simulink model "Main_Firmware_LOCAL"  (R2024b)
settings: Solver=FixedStepDiscrete  StartTime=0.0  StopTime=inf  FixedStep=sample_time  RelTol=1e-3  EnableMultiTasking=on
values from neighbouring files (symbols this model uses):
  A_f = 1.24    [Minh_Inverter_Init.m]
  C_d = 0.7041    [Minh_Inverter_Init.m]
  C_rr = 0.02    [Minh_Inverter_Init.m]
  Current_max = min(InvCurr_RMS,mCurr_RMS)*sqrt(2)    [Minh_Inverter_Init.m]
  Encoder_Offset = (PhaseA_offset/ppair)*pi/180    (= -0.785398163397)    [Minh_Inverter_Init.m]
  EPWM_F = 200000    [Minh_Inverter_Init.m]
  g = 9.8    [Minh_Inverter_Init.m]
  Inertia_z = c2d(Inertia_s, sample_time, 'zoh')    [Minh_Inverter_Init.m]
  k = 1    [Minh_Inverter_Init.m]
  lambda = 0.0375    [Minh_Inverter_Init.m]
  Ld = 0.1e-3    (= 0.0001)    [Minh_Inverter_Init.m]
  Lq = Ld    (= 0.0001)    [Minh_Inverter_Init.m]
  m = 1    [Minh_Inverter_Init.m]
  ppair = 4    [Minh_Inverter_Init.m]
  r = 0.4064/2    (= 0.2032)    [Minh_Inverter_Init.m]
  rho = 1.2    [Minh_Inverter_Init.m]
  Rs = (Rpp^2)/(Rpp*3)    (= 0.00433333333333)    [Minh_Inverter_Init.m]
  sample_time = 1/10000    (= 0.0001)    [Minh_Inverter_Init.m]
  speed_max = rpm_max*2*pi/60    (= 523.598775598)    [Minh_Inverter_Init.m]
  Torque_max = Current_max*3*lambda*ppair/2    [Minh_Inverter_Init.m]
  Voltage_max = min(V_dd,mVolt_RMS*sqrt(2))    [Minh_Inverter_Init.m]
undefined symbols (not defined in the file or in its folder): DiscIntNeverNeededParam, dspblkCoreblockFVToolHelper, gcbh, GPTRIP1SEL, TZ1
libraries: c2802xlib x8, simulink x4, slpidlib x3, spsabctodq0Lib x2, c28004xlib x1, spsdq0toabcLib x1
(part 1 of 2)
settings Model: SimulationMode=external  ExtModeTrigDuration=8  Creator=minhp  LastModifiedBy=minhp
settings SolverCC: AllowMultiTaskInputOutput=on  AutoInsertRateTranBlk=on
settings OptimizationCC: DefaultUnderspecifiedDataType=single  EnhancedBackFolding=on  PassReuseOutputArgsAs=Individual arguments  MaxStackSize=1024  OptimizeBlockOrder=speed  DifferentSizesBufferReuse=on  OptimizationCustomize=off  EfficientTunableParamExpr=on
settings DebuggingCC: SingleTaskRateTransMsg=warning  IntegerOverflowMsg=error  ParameterTunabilityLossMsg=error  IntegerSaturationMsg=error
settings HardwareCC: ProdBitPerChar=16  ProdBitPerInt=16  ProdBitPerPointer=32  ProdBitPerSizeT=32  ProdBitPerPtrDiffT=32  ProdLargestAtomicInteger=Integer  ProdLargestAtomicFloat=None  ProdWordSize=16  ProdLongLongMode=on  ProdHWDeviceType=Texas Instruments->C2000  HardwareBoardFeatureSet=SoCBlockset
settings SFSimCC: MATLABDynamicMemAlloc=off
settings RTWCC: Description=Embedded Coder  SystemTargetFile=ert.tlc  HardwareBoard=TI Piccolo F280049C LaunchPad  TemplateMakefile=ert_default_tmf  Toolchain=Texas Instruments Code Composer Studio (C2000)  CodeProfilingSaveOptions=MetricsOnly
settings CodeAppCC: ForceParamTrailComments=on  IgnoreCustomStorageClasses=off  OperatorAnnotations=on  SimulinkDataObjDesc=on  SFDataObjDesc=on  InsertBlockDesc=on
settings ERTTargetCC: CodeReplacementLibrary=TI C28x  SupportContinuousTime=on  ExtModeTransport=4  ExtModeStaticAlloc=on  ExtModeAutomaticAllocSize=off  ExtModeStaticAllocSize=5000  ExtModeMexFile=ext_xcp  ExtModeIntrfLevel=Level2 - Open  InlinedParameterPlacement=Hierarchical  DynamicArrayContainerType=coder::array

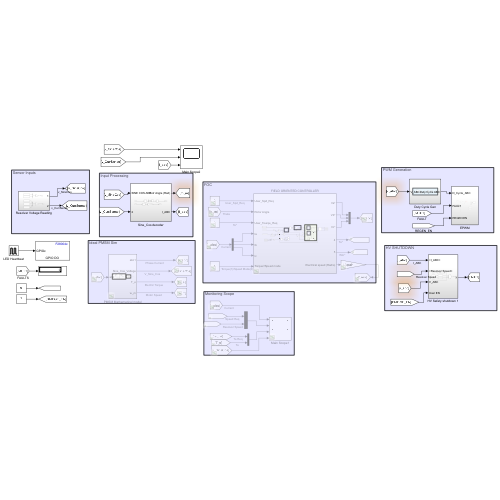
[thumbnail: Simulink's stored preview of the top-level diagram]
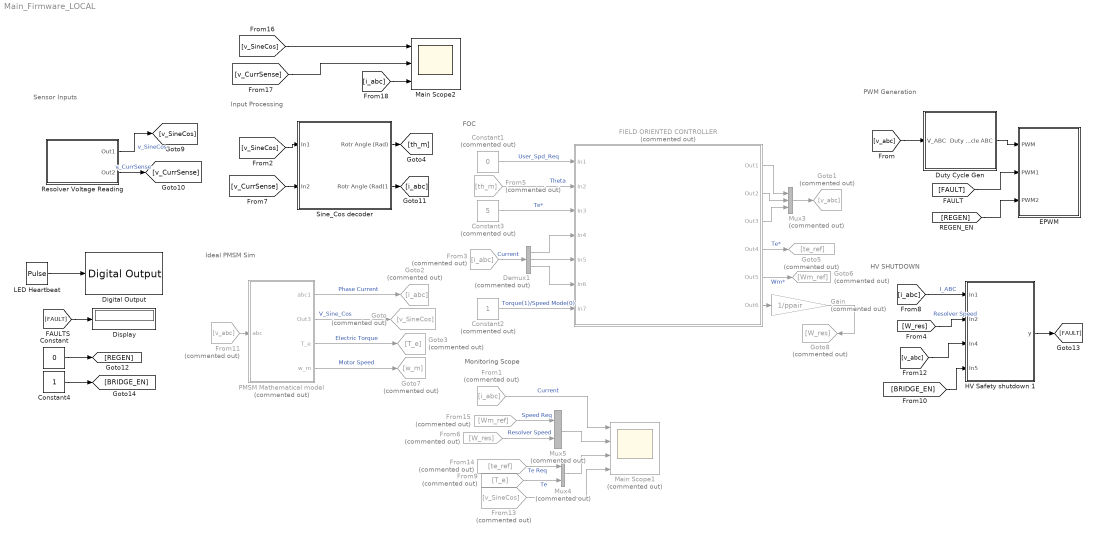
== system Main_Firmware_LOCAL ==
  note: Ideal PMSM Sim
  note: Monitoring Scope
  note: PWM Generation
  note: Input Processing
  note: FOC
  note: Sensor Inputs
  note: HV SHUTDOWN
  Constant : Constant  Value=0
  Constant1 : Constant  Commented=on  Value=0  OutDataTypeStr=single
  Constant2 : Constant  Commented=on
  Constant3 : Constant  Commented=on  Value=5  OutDataTypeStr=single
  Constant4 : Constant
  Demux1 : Demux  Commented=on  Outputs=3
  Digital Output : c28004xlib/Digital Output  GPIO_Number=GPIO16~GPIO23  GPIO_Bit0=off  GPIO_BIT0_Toggle=off  GPIO_Bit1=off  GPIO_BIT1_Toggle=off  GPIO_Bit2=off  GPIO_BIT2_Toggle=off  GPIO_Bit3=off  GPIO_BIT3_Toggle=off  GPIO_Bit4=off  GPIO_BIT4_Toggle=off  GPIO_Bit5=off  GPIO_BIT5_Toggle=off  GPIO_Bit6=off  GPIO_BIT6_Toggle=off  GPIO_Bit7=on  GPIO_BIT7_Toggle=off
  Display : Display
  Duty Cycle Gen : Subsystem
  EPWM : Subsystem
  FIELD ORIENTED CONTROLLER : Subsystem  Commented=on
  From1 : From  Commented=on  GotoTag=i_abc
  From11 : From  Commented=on  GotoTag=v_abc
  From13 : From  Commented=on  GotoTag=v_SineCos
  From14 : From  Commented=on  GotoTag=te_ref
  From15 : From  Commented=on  GotoTag=Wm_ref
  From3 : From  Commented=on  GotoTag=i_abc
  From5 : From  Commented=on  GotoTag=th_m
  From6 : From  Commented=on  GotoTag=W_res
  From9 : From  Commented=on  GotoTag=T_e
  Gain : Gain  Commented=on  Gain=1/ppair
  Goto : Goto  Commented=on  GotoTag=v_SineCos
  Goto1 : Goto  Commented=on  GotoTag=v_abc
  Goto2 : Goto  Commented=on  GotoTag=i_abc
  Goto3 : Goto  Commented=on  GotoTag=T_e
  Goto5 : Goto  Commented=on  GotoTag=te_ref
  Goto6 : Goto  Commented=on  GotoTag=Wm_ref
  Goto7 : Goto  Commented=on  GotoTag=w_m
  Goto8 : Goto  Commented=on  GotoTag=W_res
  HV Safety shutdown 1 : Subsystem
  LED Heartbeat : DiscretePulseGenerator  PulseType=Time based  Period=1  PulseWidth=50
  Main Scope1 : Scope  Commented=on  NumInputPorts=4
  Main Scope2 : Scope  NumInputPorts=3
  Mux3 : Mux  Commented=on  Inputs=3
  Mux4 : Mux  Commented=on  Inputs=2
  Mux5 : Mux  Commented=on  Inputs=2
  PMSM Mathematical model : Subsystem  Commented=on
  Resolver Voltage Reading : Subsystem
  Sine_Cos decoder : Subsystem
  wires:
  Duty Cycle Gen/1(Duty Cycle ABC) -> EPWM/1(PWM)
  PMSM Mathematical model/2(Out3) -> Goto/1  "V_Sine_Cos"
  PMSM Mathematical model/4(w_m) -> Goto7/1  "Motor Speed"
  From11/1 -> PMSM Mathematical model/1(abc)
  PMSM Mathematical model/1(abc1) -> Goto2/1  "Phase Current"
  PMSM Mathematical model/3(T_e) -> Goto3/1  "Electric Torque"
  Constant3/1 -> FIELD ORIENTED CONTROLLER/3(In3)  "Te*"
  FIELD ORIENTED CONTROLLER/1(Out1) -> Mux3/1
  FIELD ORIENTED CONTROLLER/4(Out4) -> Goto5/1  "Te*"
  FIELD ORIENTED CONTROLLER/2(Out2) -> Mux3/2
  FIELD ORIENTED CONTROLLER/3(Out3) -> Mux3/3
  From3/1 -> Demux1/1  "Current"
  From5/1 -> FIELD ORIENTED CONTROLLER/2(In2)  "Theta"
  Demux1/2 -> FIELD ORIENTED CONTROLLER/5(In5)
  Demux1/3 -> FIELD ORIENTED CONTROLLER/6(In6)
  Constant2/1 -> FIELD ORIENTED CONTROLLER/7(In7)  "Torque(1)/Speed Mode(0)"
  Demux1/1 -> FIELD ORIENTED CONTROLLER/4(In4)
  Constant1/1 -> FIELD ORIENTED CONTROLLER/1(In1)  "User_Spd_Req"
  FIELD ORIENTED CONTROLLER/5(Out5) -> Goto6/1  "Wm*"
  [v_abc] -> Duty Cycle Gen/1(V_ABC)
  From6/1 -> Mux5/2  "Resolver Speed"
  From14/1 -> Mux4/1  "Te Req"
  From9/1 -> Mux4/2  "Te"
  Mux5/1 -> Main Scope1/2
  From15/1 -> Mux5/1  "Speed Req"
  From1/1 -> Main Scope1/1  "Current"
  Mux4/1 -> Main Scope1/3
  Mux3/1 -> Goto1/1
  [v_SineCos] -> Sine_Cos decoder/1(In1)
  Sine_Cos decoder/1(Rotr Angle (Rad)) -> [th_m]
  FIELD ORIENTED CONTROLLER/6(Out6) -> Gain/1
  Gain/1 -> Goto8/1
  Resolver Voltage Reading/1(Out1) -> [v_SineCos]  "v_SineCos"
  LED Heartbeat/1 -> Digital Output/1
  Resolver Voltage Reading/2(Out2) -> [v_CurrSense]  "v_CurrSense"
  [v_CurrSense] -> Sine_Cos decoder/2(In2)
  Sine_Cos decoder/2(Rotr Angle (Rad)1) -> [i_abc]
  [FAULT] -> EPWM/2(PWM1)
  [i_abc] -> HV Safety shutdown 1/1(In1)  "I_ABC"
  HV Safety shutdown 1/1(y) -> [FAULT]
  [FAULT] -> Display/1
  [W_res] -> HV Safety shutdown 1/2(In2)  "Resolver Speed"
  [v_abc] -> HV Safety shutdown 1/3(In4)
  From13/1 -> Main Scope1/4
  [v_SineCos] -> Main Scope2/1
  [v_CurrSense] -> Main Scope2/2
  [i_abc] -> Main Scope2/3
  [REGEN] -> EPWM/3(PWM2)
  [BRIDGE_EN] -> HV Safety shutdown 1/4(In5)
  Constant/1 -> [REGEN]
  Constant4/1 -> [BRIDGE_EN]

== system Main_Firmware_LOCAL/Duty Cycle Gen ==
  note: PWM Duty Cycle Generation:
  V_ABC : Inport
  Constant7 : Constant  Value=0.5
  Gain5 : Gain  Gain=1/Voltage_max  OutDataTypeStr=single  RndMeth=Nearest
  Sampling Delay : Delay  DelayLength=1
  Saturation : Saturate  UpperLimit=95  LowerLimit=0  OutDataTypeStr=single  RndMeth=Nearest
  Sum : Sum  Inputs=|++
  Duty Cycle ABC : Outport
  wires:
  Sampling Delay/1 -> Saturation/1
  Gain5/1 -> Sum/1
  Saturation/1 -> Duty Cycle ABC/1
  V_ABC/1 -> Gain5/1
  Constant7/1 -> Sum/2
  Sum/1 -> Sampling Delay/1

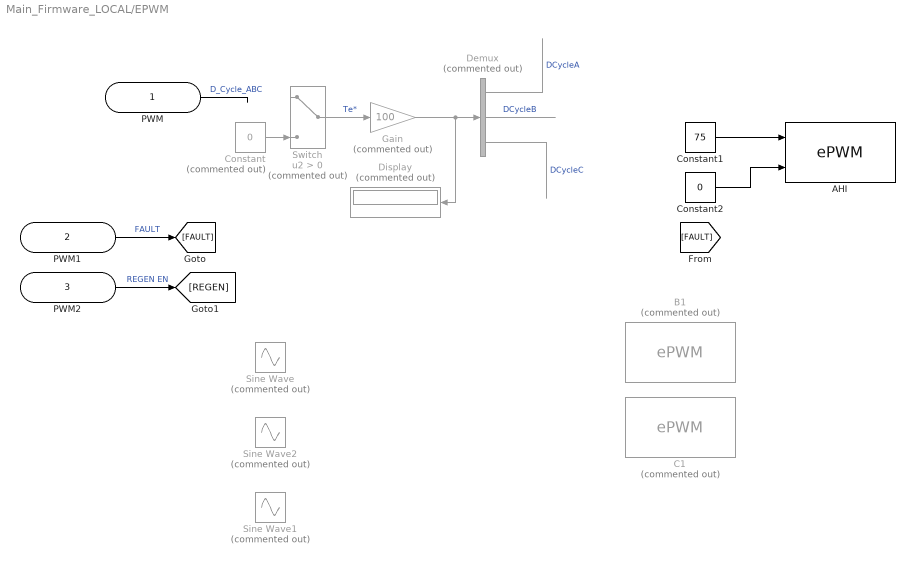
== system Main_Firmware_LOCAL/EPWM ==
  PWM : Inport
  PWM1 : Inport  Port=2
  PWM2 : Inport  Port=3
  AHI : c2802xlib/ePWM  PwmType=C2000_Type4  useModule=ePWM1  ePWMxLINKTBPRD=Not Linked  periodUnits=Seconds  timerSource=Specify via dialog  timerPeriod_clk=1/EPWM_F  timerPeriod_sec=1/EPWM_F  tbshadow=Counter equals to zero  countingMode=Up  phaseActiveEnable=Disable  phaseDirection=Count down after sync  phaseActive=0  synchronizationEnable=off  dcaevt1Sync=off  dcbevt1Sync=off  synchronizationOption=Disable  dcbevt1SyncOut=off  dcaevt1SyncOut=off  cmpdSyncOut=off  cmpcSyncOut=off  cmpbSyncOut=off  zeroSyncOut=off  swfSyncOut=off  perSynchronizationOption=Counter equals to period (CTR=PRD)  clockPrescale=1  HSclockPrescale=1  enswap=off  ePWMxAStatus=on  ePWMxAactionLogic1=Set  ePWMxAactionLogic2=Clear  ePWMxAactionLogic3=Clear  ePWMxAactionLogic4=Set  ePWMxAactionLogic5=Do nothing  ePWMxAactionLogic6=Do nothing  ePWMxACSFenable=on  ePWMxACSFvalue=Forcing low  ePWMxASFreload=Zero  ePWMxBStatus=on  ePWMxBactionLogic1=Set  ePWMxBactionLogic2=Clear  ePWMxBactionLogic3=Clear  ePWMxBactionLogic4=Do nothing  ePWMxBactionLogic5=Do nothing  ePWMxBactionLogic6=Set  ePWMxBCSFenable=off  ePWMxBCSFvalue=Forcing disable  ePWMxBSFreload=Zero  ePWNxBOutWay=off  ePWMxLINKCMPA=Not Linked  CMPAUnits=Percentages  CMPASource=Input port  CMPAValue_per=0  CMPAValue_clk=0  enCMPAshadow=Counter equals to zero (CTR=Zero)  ePWMxLINKCMPB=Not Linked  CMPBUnits=Clock cycles  CMPBSource=Specify via dialog  CMPBValue_per=50  CMPBValue_clk=32000  enCMPBshadow=Counter equals to zero (CTR=Zero)  ePWMxLINKCMPC=Not Linked  CMPCUnits=Percentages  CMPCSource=Specify via dialog  CMPCValue_per=60  CMPCValue_clk=50  enCMPCshadow=Counter equals to zero (CTR=Zero)  ePWMxLINKCMPD=Not Linked  CMPDUnits=Clock cycles  CMPDSource=Specify via dialog  CMPDValue_per=50  CMPDValue_clk=32000  enCMPDshadow=Counter equals to zero (CTR=Zero)  enableDBePWMxA=off  enableDBePWMxB=off  enhalfcycle=off  DBpolarity=Active high (AH)  DBedgeDelay=Positive  DBSource_ePWMxA=ePWMxA  DBSource_ePWMxB=ePWMxA  DBPeriodUnits=Clock cycles  DBperiodSource=Specify via dialog  REDperiod=0  FEDperiod=0  REDperiod_sec=0  FEDperiod_sec=0  LoadModeDBRED=Immediate without using shadow  LoadModeDBFED=Immediate without using shadow  adcstartModuleA=off  adcrequestEventA=First event  adcstartEventA=Digital Compare Module A Event 1 start of conversion (DCAEVT1.soc)  adcstartEventA_type2=Counter equals to zero (CTR=Zero)  adcstartModuleB=off  adcrequestEventB=First event  adcstartEventB=Counter equals to zero (CTR=Zero)  adcstartEventB_type2=Counter equals to zero (CTR=Zero)  intEn=off  intPrd=First event  intSel=Counter equals to zero (CTR=Zero)  intSel_type2=Counter equals to zero (CTR=Zero)  hrpe=off  enHRPWM=off  HRPWM_LoadMode=Counter equals to period (CTR=PRD)  HRPWM_CTLMode=Duty or Period control mode  HRPWM_EDGMode=Both edge  hrpeb=off  enHRPWMB=off  HRPWM_LoadModeB=Counter equals to zero (CTR=ZERO)  HRPWM_CTLModeB=Duty or Period control mode  HRPWM_EDGModeB=Both edge  enHRDBRED=off  enHRDBFED=off  enSFO=on  enautoconv=on  chopperEnable=off  chopperFrequency=1  chopperFirstwidth=1  chopperDuty=12.5%  tripZonesource=Specify via dialog  tzselOSHT1=off  tzselOSHT2=off  tzselOSHT3=off  tzselOSHT4=off  tzselOSHT5=off  tzselOSHT6=off  tzselOSHDCAEV1=off  tzselOSHDCBEV1=off  tzselCBC1=off  tzselCBC2=off  tzselCBC3=off  tzselCBC4=off  tzselCBC5=off  tzselCBC6=off  tzselCBCDCAEV2=off  tzselCBCDCBEV2=off  enTzOstIntr=off  enTzCbcIntr=off  enTzDCAEVT1Intr=off  enTzDCAEVT2Intr=off  enTzDCBEVT1Intr=off  enTzDCBEVT2Intr=off  tzclrCBCLatch=Counter equals to zero (CTR=Zero)  ePWMxAforced=No action  ePWMxBforced=No action  DCAEVT1forced=No action  DCBEVT1forced=No action  DCAEVT2forced=No action  DCBEVT2forced=No action  dcah=Trip Zone 1 input (TZ1)  dcal=Trip Zone 2 input (TZ2)  dcbh=Trip Zone 1 input (TZ1)  dcbl=Trip Zone 2 input (TZ2)  dcah_type2=GPTRIP1SEL/(TZ1)  dcal_type2=GPTRIP1SEL/(TZ1)  dcbh_type2=GPTRIP1SEL/(TZ1)  dcbl_type2=GPTRIP1SEL/(TZ1)  gendcaevt1=Event disabled  gendcaevt2=Event disabled  gendcbevt1=Event disabled  gendcbevt2=Event disabled  dcaevt1src=DCAEVT1 with sync  dcaevt2src=DCAEVT2 with sync  dcbevt1src=DCBEVT1 with sync  dcbevt2src=DCBEVT2 with sync  pulsesel=Counter equals to zero (CTR=Zero)  blankinv=off  blankoffset=0  blankwidth=0  evsrcsel=Filtered version of DCAEVT1 (DCAEVT1FILT)  encape=off
      settings: LibrarySourceBlock=c28004xlib/ePWM
  B1 : c2802xlib/ePWM  Commented=on  PwmType=C2000_Type4  useModule=ePWM4  ePWMxLINKTBPRD=ePWM1  periodUnits=Seconds  timerSource=Specify via dialog  timerPeriod_clk=1/EPWM_F  timerPeriod_sec=1/EPWM_F  tbshadow=Counter equals to zero  countingMode=Up  phaseActiveEnable=Disable  phaseDirection=Count down after sync  phaseActive=0  synchronizationEnable=off  dcaevt1Sync=off  dcbevt1Sync=off  synchronizationOption=Disable  dcbevt1SyncOut=off  dcaevt1SyncOut=off  cmpdSyncOut=off  cmpcSyncOut=off  cmpbSyncOut=off  zeroSyncOut=off  swfSyncOut=off  perSynchronizationOption=Counter equals to period (CTR=PRD)  clockPrescale=1  HSclockPrescale=1  enswap=off  ePWMxAStatus=on  ePWMxAactionLogic1=Set  ePWMxAactionLogic2=Clear  ePWMxAactionLogic3=Clear  ePWMxAactionLogic4=Set  ePWMxAactionLogic5=Do nothing  ePWMxAactionLogic6=Do nothing  ePWMxACSFenable=off  ePWMxACSFvalue=Forcing disable  ePWMxASFreload=Zero  ePWMxBStatus=on  ePWMxBactionLogic1=Set  ePWMxBactionLogic2=Clear  ePWMxBactionLogic3=Clear  ePWMxBactionLogic4=Do nothing  ePWMxBactionLogic5=Do nothing  ePWMxBactionLogic6=Set  ePWMxBCSFenable=off  ePWMxBCSFvalue=Forcing disable  ePWMxBSFreload=Zero  ePWNxBOutWay=off  ePWMxLINKCMPA=Not Linked  CMPAUnits=Percentages  CMPASource=Input port  CMPAValue_per=0  CMPAValue_clk=0  enCMPAshadow=Counter equals to zero (CTR=Zero)  ePWMxLINKCMPB=Not Linked  CMPBUnits=Clock cycles  CMPBSource=Specify via dialog  CMPBValue_per=50  CMPBValue_clk=32000  enCMPBshadow=Counter equals to zero (CTR=Zero)  ePWMxLINKCMPC=Not Linked  CMPCUnits=Percentages  CMPCSource=Specify via dialog  CMPCValue_per=60  CMPCValue_clk=50  enCMPCshadow=Counter equals to zero (CTR=Zero)  ePWMxLINKCMPD=Not Linked  CMPDUnits=Clock cycles  CMPDSource=Specify via dialog  CMPDValue_per=50  CMPDValue_clk=32000  enCMPDshadow=Counter equals to zero (CTR=Zero)  enableDBePWMxA=off  enableDBePWMxB=off  enhalfcycle=off  DBpolarity=Active high (AH)  DBedgeDelay=Positive  DBSource_ePWMxA=ePWMxA  DBSource_ePWMxB=ePWMxA  DBPeriodUnits=Clock cycles  DBperiodSource=Specify via dialog  REDperiod=0  FEDperiod=0  REDperiod_sec=0  FEDperiod_sec=0  LoadModeDBRED=Immediate without using shadow  LoadModeDBFED=Immediate without using shadow  adcstartModuleA=off  adcrequestEventA=First event  adcstartEventA=Digital Compare Module A Event 1 start of conversion (DCAEVT1.soc)  adcstartEventA_type2=Counter equals to zero (CTR=Zero)  adcstartModuleB=off  adcrequestEventB=First event  adcstartEventB=Counter equals to zero (CTR=Zero)  adcstartEventB_type2=Counter equals to zero (CTR=Zero)  intEn=off  intPrd=First event  intSel=Counter equals to zero (CTR=Zero)  intSel_type2=Counter equals to zero (CTR=Zero)  hrpe=off  enHRPWM=off  HRPWM_LoadMode=Counter equals to period (CTR=PRD)  HRPWM_CTLMode=Duty or Period control mode  HRPWM_EDGMode=Both edge  hrpeb=off  enHRPWMB=off  HRPWM_LoadModeB=Counter equals to zero (CTR=ZERO)  HRPWM_CTLModeB=Duty or Period control mode  HRPWM_EDGModeB=Both edge  enHRDBRED=off  enHRDBFED=off  enSFO=on  enautoconv=on  chopperEnable=off  chopperFrequency=1  chopperFirstwidth=1  chopperDuty=12.5%  tripZonesource=Specify via dialog  tzselOSHT1=off  tzselOSHT2=off  tzselOSHT3=off  tzselOSHT4=off  tzselOSHT5=off  tzselOSHT6=off  tzselOSHDCAEV1=off  tzselOSHDCBEV1=off  tzselCBC1=off  tzselCBC2=off  tzselCBC3=off  tzselCBC4=off  tzselCBC5=off  tzselCBC6=off  tzselCBCDCAEV2=off  tzselCBCDCBEV2=off  enTzOstIntr=off  enTzCbcIntr=off  enTzDCAEVT1Intr=off  enTzDCAEVT2Intr=off  enTzDCBEVT1Intr=off  enTzDCBEVT2Intr=off  tzclrCBCLatch=Counter equals to zero (CTR=Zero)  ePWMxAforced=No action  ePWMxBforced=No action  DCAEVT1forced=No action  DCBEVT1forced=No action  DCAEVT2forced=No action  DCBEVT2forced=No action  dcah=Trip Zone 1 input (TZ1)  dcal=Trip Zone 2 input (TZ2)  dcbh=Trip Zone 1 input (TZ1)  dcbl=Trip Zone 2 input (TZ2)  dcah_type2=GPTRIP1SEL/(TZ1)  dcal_type2=GPTRIP1SEL/(TZ1)  dcbh_type2=GPTRIP1SEL/(TZ1)  dcbl_type2=GPTRIP1SEL/(TZ1)  gendcaevt1=Event disabled  gendcaevt2=Event disabled  gendcbevt1=Event disabled  gendcbevt2=Event disabled  dcaevt1src=DCAEVT1 with sync  dcaevt2src=DCAEVT2 with sync  dcbevt1src=DCBEVT1 with sync  dcbevt2src=DCBEVT2 with sync  pulsesel=Counter equals to zero (CTR=Zero)  blankinv=off  blankoffset=0  blankwidth=0  evsrcsel=Filtered version of DCAEVT1 (DCAEVT1FILT)  encape=off
      settings: LibrarySourceBlock=c28004xlib/ePWM
  C1 : c2802xlib/ePWM  Commented=on  PwmType=C2000_Type4  useModule=ePWM2  ePWMxLINKTBPRD=ePWM1  periodUnits=Seconds  timerSource=Specify via dialog  timerPeriod_clk=1/EPWM_F  timerPeriod_sec=1/EPWM_F  tbshadow=Counter equals to zero  countingMode=Up  phaseActiveEnable=Disable  phaseDirection=Count down after sync  phaseActive=0  synchronizationEnable=off  dcaevt1Sync=off  dcbevt1Sync=off  synchronizationOption=Disable  dcbevt1SyncOut=off  dcaevt1SyncOut=off  cmpdSyncOut=off  cmpcSyncOut=off  cmpbSyncOut=off  zeroSyncOut=off  swfSyncOut=off  perSynchronizationOption=Counter equals to period (CTR=PRD)  clockPrescale=1  HSclockPrescale=1  enswap=off  ePWMxAStatus=on  ePWMxAactionLogic1=Set  ePWMxAactionLogic2=Clear  ePWMxAactionLogic3=Clear  ePWMxAactionLogic4=Set  ePWMxAactionLogic5=Do nothing  ePWMxAactionLogic6=Do nothing  ePWMxACSFenable=off  ePWMxACSFvalue=Forcing disable  ePWMxASFreload=Zero  ePWMxBStatus=on  ePWMxBactionLogic1=Set  ePWMxBactionLogic2=Clear  ePWMxBactionLogic3=Clear  ePWMxBactionLogic4=Do nothing  ePWMxBactionLogic5=Do nothing  ePWMxBactionLogic6=Set  ePWMxBCSFenable=off  ePWMxBCSFvalue=Forcing disable  ePWMxBSFreload=Zero  ePWNxBOutWay=off  ePWMxLINKCMPA=Not Linked  CMPAUnits=Percentages  CMPASource=Input port  CMPAValue_per=0  CMPAValue_clk=0  enCMPAshadow=Counter equals to zero (CTR=Zero)  ePWMxLINKCMPB=Not Linked  CMPBUnits=Clock cycles  CMPBSource=Specify via dialog  CMPBValue_per=50  CMPBValue_clk=32000  enCMPBshadow=Counter equals to zero (CTR=Zero)  ePWMxLINKCMPC=Not Linked  CMPCUnits=Percentages  CMPCSource=Specify via dialog  CMPCValue_per=60  CMPCValue_clk=50  enCMPCshadow=Counter equals to zero (CTR=Zero)  ePWMxLINKCMPD=Not Linked  CMPDUnits=Clock cycles  CMPDSource=Specify via dialog  CMPDValue_per=50  CMPDValue_clk=32000  enCMPDshadow=Counter equals to zero (CTR=Zero)  enableDBePWMxA=off  enableDBePWMxB=off  enhalfcycle=off  DBpolarity=Active high (AH)  DBedgeDelay=Positive  DBSource_ePWMxA=ePWMxA  DBSource_ePWMxB=ePWMxA  DBPeriodUnits=Clock cycles  DBperiodSource=Specify via dialog  REDperiod=0  FEDperiod=0  REDperiod_sec=0  FEDperiod_sec=0  LoadModeDBRED=Immediate without using shadow  LoadModeDBFED=Immediate without using shadow  adcstartModuleA=off  adcrequestEventA=First event  adcstartEventA=Digital Compare Module A Event 1 start of conversion (DCAEVT1.soc)  adcstartEventA_type2=Counter equals to zero (CTR=Zero)  adcstartModuleB=off  adcrequestEventB=First event  adcstartEventB=Counter equals to zero (CTR=Zero)  adcstartEventB_type2=Counter equals to zero (CTR=Zero)  intEn=off  intPrd=First event  intSel=Counter equals to zero (CTR=Zero)  intSel_type2=Counter equals to zero (CTR=Zero)  hrpe=off  enHRPWM=off  HRPWM_LoadMode=Counter equals to period (CTR=PRD)  HRPWM_CTLMode=Duty or Period control mode  HRPWM_EDGMode=Both edge  hrpeb=off  enHRPWMB=off  HRPWM_LoadModeB=Counter equals to zero (CTR=ZERO)  HRPWM_CTLModeB=Duty or Period control mode  HRPWM_EDGModeB=Both edge  enHRDBRED=off  enHRDBFED=off  enSFO=on  enautoconv=on  chopperEnable=off  chopperFrequency=1  chopperFirstwidth=1  chopperDuty=12.5%  tripZonesource=Specify via dialog  tzselOSHT1=off  tzselOSHT2=off  tzselOSHT3=off  tzselOSHT4=off  tzselOSHT5=off  tzselOSHT6=off  tzselOSHDCAEV1=off  tzselOSHDCBEV1=off  tzselCBC1=off  tzselCBC2=off  tzselCBC3=off  tzselCBC4=off  tzselCBC5=off  tzselCBC6=off  tzselCBCDCAEV2=off  tzselCBCDCBEV2=off  enTzOstIntr=off  enTzCbcIntr=off  enTzDCAEVT1Intr=off  enTzDCAEVT2Intr=off  enTzDCBEVT1Intr=off  enTzDCBEVT2Intr=off  tzclrCBCLatch=Counter equals to zero (CTR=Zero)  ePWMxAforced=No action  ePWMxBforced=No action  DCAEVT1forced=No action  DCBEVT1forced=No action  DCAEVT2forced=No action  DCBEVT2forced=No action  dcah=Trip Zone 1 input (TZ1)  dcal=Trip Zone 2 input (TZ2)  dcbh=Trip Zone 1 input (TZ1)  dcbl=Trip Zone 2 input (TZ2)  dcah_type2=GPTRIP1SEL/(TZ1)  dcal_type2=GPTRIP1SEL/(TZ1)  dcbh_type2=GPTRIP1SEL/(TZ1)  dcbl_type2=GPTRIP1SEL/(TZ1)  gendcaevt1=Event disabled  gendcaevt2=Event disabled  gendcbevt1=Event disabled  gendcbevt2=Event disabled  dcaevt1src=DCAEVT1 with sync  dcaevt2src=DCAEVT2 with sync  dcbevt1src=DCBEVT1 with sync  dcbevt2src=DCBEVT2 with sync  pulsesel=Counter equals to zero (CTR=Zero)  blankinv=off  blankoffset=0  blankwidth=0  evsrcsel=Filtered version of DCAEVT1 (DCAEVT1FILT)  encape=off
      settings: LibrarySourceBlock=c28004xlib/ePWM
  Constant : Constant  Commented=on  Value=0
  Constant1 : Constant  Value=75
  Constant2 : Constant  Value=0
  Demux : Demux  Commented=on  Outputs=3
  Display : Display  Commented=on
  Gain : Gain  Commented=on  Gain=100
  Sine Wave : Sin  Commented=on  Amplitude=50  Bias=50  Frequency=0.1*2*pi  SampleTime=0
  Sine Wave1 : Sin  Commented=on  Amplitude=50  Bias=50  Frequency=0.1*2*pi  Phase=-2*pi/3  SampleTime=0
  Sine Wave2 : Sin  Commented=on  Amplitude=50  Bias=50  Frequency=0.1*2*pi  Phase=2*pi/3  SampleTime=0
  Switch : Switch  Commented=on  Criteria=u2 > Threshold  OutDataTypeStr=single  SaturateOnIntegerOverflow=off  InputSameDT=off
  wires:
  Demux/2 -> ?  "DCycleB"
  Demux/3 -> ?  "DCycleC"
  PWM/1 -> ?  "D_Cycle_ABC"
  Demux/1 -> ?  "DCycleA"
  Gain/1 -> Demux/1, Display/1
  Switch/1 -> Gain/1  "Te*"
  PWM1/1 -> [FAULT]  "FAULT"
  Constant/1 -> Switch/3
  Constant1/1 -> AHI/1
  Constant2/1 -> AHI/2
  PWM2/1 -> [REGEN]  "REGEN EN"

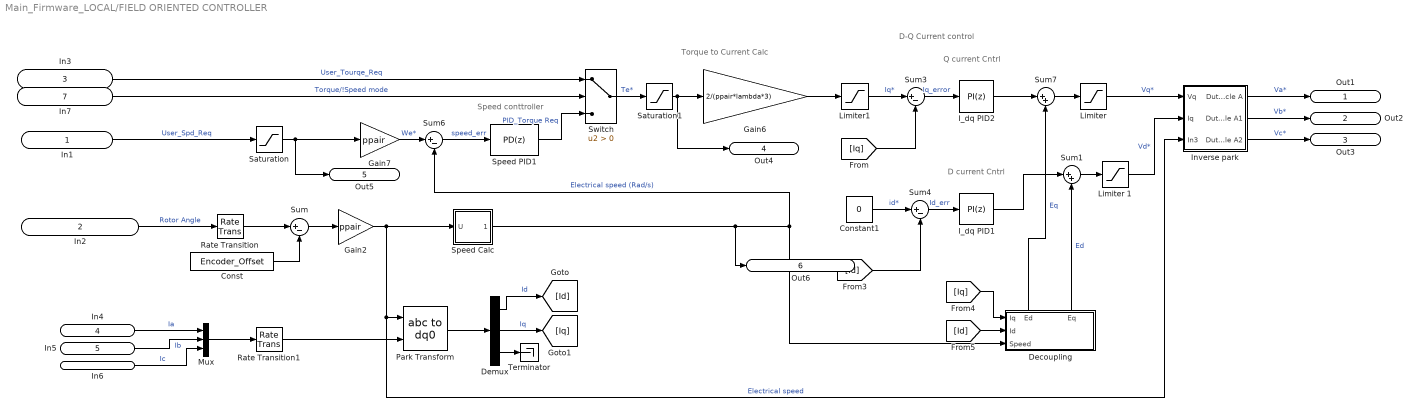
== system Main_Firmware_LOCAL/FIELD ORIENTED CONTROLLER ==
  note: Torque to Current Calc
  note: Speed conttroller
  note: D current
      | Cntrl
  note: D-Q Current control
  note: Q current
      | Cntrl
  In1 : Inport
  In2 : Inport  Port=2
  In3 : Inport  Port=3
  In4 : Inport  Port=4
  In5 : Inport  Port=5
  In6 : Inport  Port=6
  In7 : Inport  Port=7
  Const : Constant  Value=Encoder_Offset
  Constant1 : Constant  Value=0
  Decoupling : Subsystem
      settings: PortSchema="{\"entries\":[{\"content\":{\"sides\":[{\"content\":{\"connectorIds\":[\"In1\",\"In2\",\"In3\"]},\"type\":\"ConnectorPlacement.EquallySpacedRectSide\",\"uuid\":\"5f512ccb-8595-4499-a419-e995908cd1f5\"},{\"content\":{\"side\":\"RIGHT\"},\"type\":\"ConnectorPlacement.EquallySpacedRectSide\",\"uuid\":\"2a1de219-597a-4818-9587-d28590d7f25d\"},{\"content\":{\"connectorIds\":[\"Out1\",\"Out2\"],\"side\":\"TOP\"},\"type\":\"ConnectorPlacement.EquallySpacedRectSide\",\"uuid\":\"87b053a8-3806-4156-bae7-a97f33c02d51\"}]},\"type\":\"ConnectorPlacement.EquallySpacedConnector\",\"uuid\":\"5d9f8914-d3c5-4fbe-94a4-f1d2e0d8a5f7\"}],\"packageUris\":[\"http://schema.mathworks.com/mf0/Connector/R2020b\"],\"version\":\"1.0\"}"
  Demux : Demux  Outputs=3
  Gain2 : Gain  Gain=ppair  OutDataTypeStr=single  RndMeth=Nearest
  Gain6 : Gain  Gain=2/(ppair*lambda*3)  OutDataTypeStr=single  RndMeth=Nearest
  Gain7 : Gain  Gain=ppair  OutDataTypeStr=single  RndMeth=Nearest
  I_dq PID1 : slpidlib/PID Controller  Controller=PI  Form=Parallel  TimeDomain=Discrete-time  UseExternalTs=off  SampleTime=-1  IntegratorMethod=Forward Euler  FilterMethod=Forward Euler  ControllerParametersSource=internal  P=0.216674080570424  I=8.23559930371868  UseKiTs=off  D=2.81416629288768e-05  UseExternalDerivativeSource=off  N=4271.19819316481  UseFilter=on  TunerSelectOption=Transfer Function Based (PID Tuner App)  InitialConditionSource=internal  InitialConditionForIntegrator=0  InitialConditionForFilter=0  DifferentiatorICPrevScaledInput=0  ExternalReset=none  TrackingMode=off  Kt=1  LimitOutput=on  SatLimitsSource=internal  UpperSaturationLimit=Voltage_max  LowerSaturationLimit=-Voltage_max  LinearizeAsGain=off  AntiWindupMode=none  Kb=1  LimitIntegrator=on  UpperIntegratorSaturationLimit=Voltage_max  LowerIntegratorSaturationLimit=-Voltage_max  RndMeth=Nearest  PGainOutDataTypeStr=single  PProdOutDataTypeStr=single  POutMin=[]  POutMax=[]  IGainOutDataTypeStr=single  IProdOutDataTypeStr=single  IOutMin=[]  IOutMax=[]  DOutMin=[]  DOutMax=[]  NOutMin=[]  NOutMax=[]  SumOutDataTypeStr=single  SumOutMin=[]  SumOutMax=[]  SaturationOutDataTypeStr=single  SaturationOutMin=[]  SaturationOutMax=[]  PParamMin=[]  PParamMax=[]  IParamMin=[]  IParamMax=[]  DParamMin=[]  DParamMax=[]  NParamMin=[]  NParamMax=[]  KbParamMin=[]  KbParamMax=[]  KtParamMin=[]  KtParamMax=[]  KbOutMin=[]  KbOutMax=[]  KtOutMin=[]  KtOutMax=[]  IntegratorOutMin=[]  IntegratorOutMax=[]  FilterOutMin=[]  FilterOutMax=[]  SumI1OutMin=[]  SumI1OutMax=[]  SumI2OutMin=[]  SumI2OutMax=[]  SumI3OutMin=[]  SumI3OutMax=[]  SumI4OutMin=[]  SumI4OutMax=[]  SumDOutMin=[]  SumDOutMax=[]  DifferentiatorOutMin=[]  DifferentiatorOutMax=[]  FilterDiffOutCoefMin=[]  FilterDiffOutCoefMax=[]  ReciprocalOutMin=[]  ReciprocalOutMax=[]  SumDenOutMin=[]  SumDenOutMax=[]  SumNumOutMin=[]  SumNumOutMax=[]  DivideOutMin=[]  DivideOutMax=[]  UdiffTsProdOutMin=[]  UdiffTsProdOutMax=[]  NTsProdOutMin=[]  NTsProdOutMax=[]  UintegralTsProdOutMin=[]  UintegralTsProdOutMax=[]  UngainTsProdOutMin=[]  UngainTsProdOutMax=[]  ClampingZeroOutDataTypeStr=Inherit: Inherit via back propagation  ClampingZeroOutMin=[]  ClampingZeroOutMax=[]  FilterDenConstantOutDataTypeStr=Inherit: Inherit via back propagation  FilterDenConstantOutMin=[]  FilterDenConstantOutMax=[]  PCopyOutDataTypeStr=Inherit: Inherit via back propagation  PCopyOutMin=[]  PCopyOutMax=[]  NCopyOutDataTypeStr=Inherit: Inherit via back propagation  NCopyOutMin=[]  NCopyOutMax=[]  IntegratorContinuousStateAttributes=''  IntegratorStateMustResolveToSignalObject=off  IntegratorRTWStateStorageClass=Auto  FilterContinuousStateAttributes=''  FilterStateMustResolveToSignalObject=off  FilterRTWStateStorageClass=Auto  ParallelPVariant=InternalParameters  IdealPVariant=Disabled  IVariant=InternalParameters  DVariant=Disabled  IntegratorVariant=Discrete  SatVariant=Enabled  AWVariant=Passthrough  PCopyVariant=Disabled  TRVariant=Disabled  FdbkBlocksVariant=Forward  IdealPFdbkVariant=Disabled  SatFdbkVariant=Disabled  DerivativeFilterVariant=Disabled  NVariant=Disabled  NCopyVariant=Disabled_SignalSpec  FilterICVariant=Disabled  IntegratorICVariant=InternalICs  ExternalResetVariant=Disabled  TRSumVariant=Passthrough  SumFdbkVariant=Disabled  SumVariant=Sum_PI  TsampFilterVariant=InternalTs  TsampNgainVariant=Passthrough  TsampIntegralVariant=Disabled_SignalSpec  ExternalSaturationOutDataTypeStr=Inherit: Same as second input  DerivativeSourceVariant=Disabled  PreIntVariant=InternalPreInt
  I_dq PID2 : slpidlib/PID Controller  Controller=PI  Form=Parallel  TimeDomain=Discrete-time  UseExternalTs=off  SampleTime=-1  IntegratorMethod=Forward Euler  FilterMethod=Forward Euler  ControllerParametersSource=internal  P=0.216674080570424  I=8.23559930371868  UseKiTs=off  D=2.81416629288768e-05  UseExternalDerivativeSource=off  N=4271.19819316481  UseFilter=on  TunerSelectOption=Transfer Function Based (PID Tuner App)  InitialConditionSource=internal  InitialConditionForIntegrator=0  InitialConditionForFilter=0  DifferentiatorICPrevScaledInput=0  ExternalReset=none  TrackingMode=off  Kt=1  LimitOutput=on  SatLimitsSource=internal  UpperSaturationLimit=Voltage_max  LowerSaturationLimit=-Voltage_max  LinearizeAsGain=off  AntiWindupMode=none  Kb=1  LimitIntegrator=on  UpperIntegratorSaturationLimit=Voltage_max  LowerIntegratorSaturationLimit=-Voltage_max  RndMeth=Nearest  PGainOutDataTypeStr=single  PProdOutDataTypeStr=single  POutMin=[]  POutMax=[]  IGainOutDataTypeStr=single  IProdOutDataTypeStr=single  IOutMin=[]  IOutMax=[]  DOutMin=[]  DOutMax=[]  NOutMin=[]  NOutMax=[]  SumOutDataTypeStr=single  SumOutMin=[]  SumOutMax=[]  SaturationOutDataTypeStr=single  SaturationOutMin=[]  SaturationOutMax=[]  PParamMin=[]  PParamMax=[]  IParamMin=[]  IParamMax=[]  DParamMin=[]  DParamMax=[]  NParamMin=[]  NParamMax=[]  KbParamMin=[]  KbParamMax=[]  KtParamMin=[]  KtParamMax=[]  KbOutMin=[]  KbOutMax=[]  KtOutMin=[]  KtOutMax=[]  IntegratorOutMin=[]  IntegratorOutMax=[]  FilterOutMin=[]  FilterOutMax=[]  SumI1OutMin=[]  SumI1OutMax=[]  SumI2OutMin=[]  SumI2OutMax=[]  SumI3OutMin=[]  SumI3OutMax=[]  SumI4OutMin=[]  SumI4OutMax=[]  SumDOutMin=[]  SumDOutMax=[]  DifferentiatorOutMin=[]  DifferentiatorOutMax=[]  FilterDiffOutCoefMin=[]  FilterDiffOutCoefMax=[]  ReciprocalOutMin=[]  ReciprocalOutMax=[]  SumDenOutMin=[]  SumDenOutMax=[]  SumNumOutMin=[]  SumNumOutMax=[]  DivideOutMin=[]  DivideOutMax=[]  UdiffTsProdOutMin=[]  UdiffTsProdOutMax=[]  NTsProdOutMin=[]  NTsProdOutMax=[]  UintegralTsProdOutMin=[]  UintegralTsProdOutMax=[]  UngainTsProdOutMin=[]  UngainTsProdOutMax=[]  ClampingZeroOutDataTypeStr=Inherit: Inherit via back propagation  ClampingZeroOutMin=[]  ClampingZeroOutMax=[]  FilterDenConstantOutDataTypeStr=Inherit: Inherit via back propagation  FilterDenConstantOutMin=[]  FilterDenConstantOutMax=[]  PCopyOutDataTypeStr=Inherit: Inherit via back propagation  PCopyOutMin=[]  PCopyOutMax=[]  NCopyOutDataTypeStr=Inherit: Inherit via back propagation  NCopyOutMin=[]  NCopyOutMax=[]  IntegratorContinuousStateAttributes=''  IntegratorStateMustResolveToSignalObject=off  IntegratorRTWStateStorageClass=Auto  FilterContinuousStateAttributes=''  FilterStateMustResolveToSignalObject=off  FilterRTWStateStorageClass=Auto  ParallelPVariant=InternalParameters  IdealPVariant=Disabled  IVariant=InternalParameters  DVariant=Disabled  IntegratorVariant=Discrete  SatVariant=Enabled  AWVariant=Passthrough  PCopyVariant=Disabled  TRVariant=Disabled  FdbkBlocksVariant=Forward  IdealPFdbkVariant=Disabled  SatFdbkVariant=Disabled  DerivativeFilterVariant=Disabled  NVariant=Disabled  NCopyVariant=Disabled_SignalSpec  FilterICVariant=Disabled  IntegratorICVariant=InternalICs  ExternalResetVariant=Disabled  TRSumVariant=Passthrough  SumFdbkVariant=Disabled  SumVariant=Sum_PI  TsampFilterVariant=InternalTs  TsampNgainVariant=Passthrough  TsampIntegralVariant=Disabled_SignalSpec  ExternalSaturationOutDataTypeStr=Inherit: Same as second input  DerivativeSourceVariant=Disabled  PreIntVariant=InternalPreInt
  Inverse park : Subsystem
  Limiter : Saturate  UpperLimit=Voltage_max  LowerLimit=0  LinearizeAsGain=off
  Limiter 1 : Saturate  UpperLimit=Voltage_max  LowerLimit=0  LinearizeAsGain=off
  Limiter1 : Saturate  UpperLimit=Current_max  LowerLimit=-Current_max  LinearizeAsGain=off
  Mux : Mux  Inputs=3
  Park Transform : spsabctodq0Lib/abc to dq0  Alignment=Aligned with phase A axis
  Rate Transition : RateTransition  OutPortSampleTime=sample_time
  Rate Transition1 : RateTransition  OutPortSampleTime=sample_time
  Saturation : Saturate  UpperLimit=speed_max  LowerLimit=-speed_max
  Saturation1 : Saturate  UpperLimit=Torque_max  LowerLimit=-Torque_max  OutDataTypeStr=single  RndMeth=Nearest
  Speed Calc : Subsystem
  Speed PID1 : slpidlib/PID Controller  Controller=PD  Form=Parallel  TimeDomain=Discrete-time  UseExternalTs=off  SampleTime=-1  IntegratorMethod=Forward Euler  FilterMethod=Forward Euler  ControllerParametersSource=internal  P=20.6545195236646  I=640.266262711417  UseKiTs=off  D=0.00205517598679868  UseExternalDerivativeSource=off  N=100.498329175013  UseFilter=on  TunerSelectOption=Transfer Function Based (PID Tuner App)  InitialConditionSource=internal  InitialConditionForIntegrator=0  InitialConditionForFilter=0  DifferentiatorICPrevScaledInput=0  ExternalReset=none  TrackingMode=off  Kt=1  LimitOutput=on  SatLimitsSource=internal  UpperSaturationLimit=Torque_max  LowerSaturationLimit=-Torque_max  LinearizeAsGain=off  AntiWindupMode=none  Kb=1  LimitIntegrator=on  UpperIntegratorSaturationLimit=Torque_max  LowerIntegratorSaturationLimit=-Torque_max  RndMeth=Nearest  PGainOutDataTypeStr=single  PProdOutDataTypeStr=single  POutMin=[]  POutMax=[]  IOutMin=[]  IOutMax=[]  DGainOutDataTypeStr=single  DProdOutDataTypeStr=single  DOutMin=[]  DOutMax=[]  NGainOutDataTypeStr=single  NProdOutDataTypeStr=single  NOutMin=[]  NOutMax=[]  SumOutDataTypeStr=single  SumOutMin=[]  SumOutMax=[]  SaturationOutDataTypeStr=single  SaturationOutMin=[]  SaturationOutMax=[]  PParamMin=[]  PParamMax=[]  IParamMin=[]  IParamMax=[]  DParamMin=[]  DParamMax=[]  NParamMin=[]  NParamMax=[]  KbParamMin=[]  KbParamMax=[]  KtParamMin=[]  KtParamMax=[]  KbOutMin=[]  KbOutMax=[]  KtOutMin=[]  KtOutMax=[]  IntegratorOutMin=[]  IntegratorOutMax=[]  FilterOutMin=[]  FilterOutMax=[]  SumI1OutMin=[]  SumI1OutMax=[]  SumI2OutMin=[]  SumI2OutMax=[]  SumI3OutMin=[]  SumI3OutMax=[]  SumI4OutMin=[]  SumI4OutMax=[]  SumDOutMin=[]  SumDOutMax=[]  DifferentiatorOutMin=[]  DifferentiatorOutMax=[]  FilterDiffOutCoefMin=[]  FilterDiffOutCoefMax=[]  ReciprocalOutMin=[]  ReciprocalOutMax=[]  SumDenOutMin=[]  SumDenOutMax=[]  SumNumOutMin=[]  SumNumOutMax=[]  DivideOutMin=[]  DivideOutMax=[]  UdiffTsProdOutMin=[]  UdiffTsProdOutMax=[]  NTsProdOutMin=[]  NTsProdOutMax=[]  UintegralTsProdOutMin=[]  UintegralTsProdOutMax=[]  UngainTsProdOutMin=[]  UngainTsProdOutMax=[]  ClampingZeroOutDataTypeStr=Inherit: Inherit via back propagation  ClampingZeroOutMin=[]  ClampingZeroOutMax=[]  FilterDenConstantOutDataTypeStr=Inherit: Inherit via back propagation  FilterDenConstantOutMin=[]  FilterDenConstantOutMax=[]  PCopyOutDataTypeStr=Inherit: Inherit via back propagation  PCopyOutMin=[]  PCopyOutMax=[]  NCopyOutDataTypeStr=Inherit: Inherit via back propagation  NCopyOutMin=[]  NCopyOutMax=[]  IntegratorContinuousStateAttributes=''  IntegratorStateMustResolveToSignalObject=off  IntegratorRTWStateStorageClass=Auto  FilterContinuousStateAttributes=''  FilterStateMustResolveToSignalObject=off  FilterRTWStateStorageClass=Auto  ParallelPVariant=InternalParameters  IdealPVariant=Disabled  IVariant=Disabled  DVariant=InternalParameters  IntegratorVariant=Disabled  SatVariant=Enabled  AWVariant=Disabled  PCopyVariant=Disabled  TRVariant=Disabled  FdbkBlocksVariant=Forward  IdealPFdbkVariant=Disabled  SatFdbkVariant=Disabled  DerivativeFilterVariant=ForwardEulerFilter  NVariant=InternalParameters  NCopyVariant=Disabled  FilterICVariant=InternalICsFilter  IntegratorICVariant=Disabled  ExternalResetVariant=Disabled  TRSumVariant=Passthrough  SumFdbkVariant=Disabled  SumVariant=Sum_PD  TsampFilterVariant=InternalTs  TsampNgainVariant=Passthrough  TsampIntegralVariant=Disabled_SignalSpec  ExternalSaturationOutDataTypeStr=Inherit: Same as second input  DerivativeSourceVariant=ErrorSignal  PreIntVariant=InternalPreInt
  Sum : Sum  Inputs=|+-  OutDataTypeStr=single  AccumDataTypeStr=single  RndMeth=Nearest
  Sum1 : Sum  Inputs=|++
  Sum3 : Sum  Inputs=|+-
  Sum4 : Sum  Inputs=|+-
  Sum6 : Sum  Inputs=|+-  OutDataTypeStr=single  RndMeth=Nearest
  Sum7 : Sum  Inputs=|++
  Switch : Switch  Criteria=u2 > Threshold  OutDataTypeStr=single  SaturateOnIntegerOverflow=off  InputSameDT=off
  Terminator : Terminator
  Out1 : Outport
  Out2 : Outport  Port=2
  Out3 : Outport  Port=3
  Out4 : Outport  Port=4
  Out5 : Outport  Port=5
  Out6 : Outport  Port=6
  wires:
  In5/1 -> Mux/2  "Ib"
  In6/1 -> Mux/3  "Ic"
  I_dq PID1/1 -> Sum1/1
  [Id] -> Sum4/2
  Demux/2 -> [Iq]  "Iq"
  Inverse park/1(Duty Cycle A) -> Out1/1  "Va*"
  I_dq PID2/1 -> Sum7/1
  Inverse park/3(Duty Cycle A2) -> Out3/1  "Vc*"
  [Iq] -> Sum3/2
  Demux/1 -> [Id]  "Id"
  [Iq] -> Decoupling/1(Iq)
  Demux/3 -> Terminator/1
  Sum3/1 -> I_dq PID2/1  "Iq_error"
  Decoupling/2(Eq) -> Sum1/2  "Ed"
  Sum7/1 -> Limiter/1
  Limiter 1/1 -> Inverse park/2(Iq)  "Vd*"
  Decoupling/1(Ed) -> Sum7/2  "Eq"
  In1/1 -> Saturation/1  "User_Spd_Req"
  Inverse park/2(Duty Cycle A1) -> Out2/1  "Vb*"
  Sum4/1 -> I_dq PID1/1  "Id_err"
  Sum1/1 -> Limiter 1/1
  Sum6/1 -> Speed PID1/1  "speed_err"
  Constant1/1 -> Sum4/1  "id*"
  Speed PID1/1 -> Switch/3  "PID_Torque Req"
  [Id] -> Decoupling/2(Id)
  In4/1 -> Mux/1  "Ia"
  Limiter/1 -> Inverse park/1(Vq)  "Vq*"
  Gain6/1 -> Limiter1/1
  In3/1 -> Switch/1  "User_Tourqe_Req"
  Park Transform/1 -> Demux/1
  In2/1 -> Rate Transition/1  "Rotor Angle"
  In7/1 -> Switch/2  "Torque/!Speed mode"
  Limiter1/1 -> Sum3/1  "Iq*"
  Gain7/1 -> Sum6/1  "We*"
  Gain2/1 -> Inverse park/3(In3), Park Transform/2, Speed Calc/1(U)  "Electrical speed"
  Const/1 -> Sum/2
  Sum/1 -> Gain2/1
  Mux/1 -> Rate Transition1/1
  Switch/1 -> Saturation1/1  "Te*"
  Saturation/1 -> Gain7/1, Out5/1
  Rate Transition/1 -> Sum/1
  Rate Transition1/1 -> Park Transform/1
  Saturation1/1 -> Out4/1, Gain6/1
  Speed Calc/1(Out1) -> Out6/1, Sum6/2, Decoupling/3(Speed)  "Electrical speed (Rad/s)"

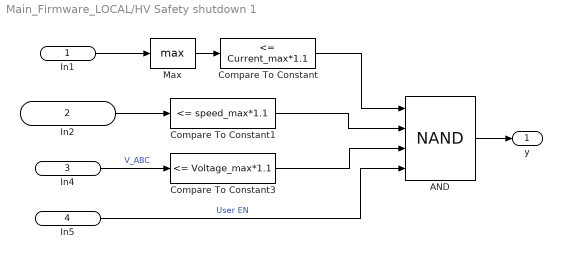
== system Main_Firmware_LOCAL/HV Safety shutdown 1 ==
  In1 : Inport
  In2 : Inport  Port=2
  In4 : Inport  Port=3
  In5 : Inport  Port=4
  AND : Logic  Operator=NAND  Inputs=4  IconShape=distinctive  AllPortsSameDT=off  OutDataTypeStr=boolean
  Compare To Constant : simulink/Logic and Bit Operations/Compare To Constant  relop=<=  const=Current_max*1.1  OutDataTypeStr=boolean
  Compare To Constant1 : simulink/Logic and Bit Operations/Compare To Constant  relop=<=  const=speed_max*1.1  OutDataTypeStr=boolean
  Compare To Constant3 : simulink/Logic and Bit Operations/Compare To Constant  relop=<=  const=Voltage_max*1.1  OutDataTypeStr=boolean
  Max : MinMax  Function=max
  y : Outport
  wires:
  Max/1 -> Compare To Constant/1
  In1/1 -> Max/1
  Compare To Constant/1 -> AND/1
  In2/1 -> Compare To Constant1/1
  Compare To Constant1/1 -> AND/2
  AND/1 -> y/1
  In4/1 -> Compare To Constant3/1  "V_ABC"
  Compare To Constant3/1 -> AND/3
  In5/1 -> AND/4  "User EN"

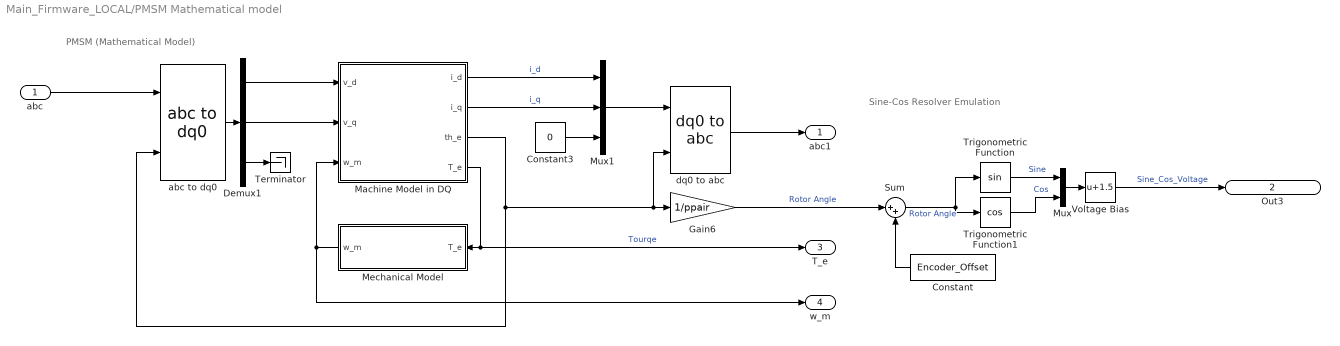
== system Main_Firmware_LOCAL/PMSM Mathematical model ==
  note: PMSM (Mathematical Model)
  note: Sine-Cos Resolver Emulation
  abc : Inport
  Constant : Constant  Value=Encoder_Offset  OutDataTypeStr=single
  Constant3 : Constant  Value=0  OutDataTypeStr=single
  Demux1 : Demux  Outputs=3
  Gain6 : Gain  Gain=1/ppair  OutDataTypeStr=single  RndMeth=Nearest
  Machine Model in DQ : Subsystem
  Mechanical Model : Subsystem
  Mux : Mux  Inputs=2
  Mux1 : Mux  Inputs=3
  Sum : Sum  Inputs=|++  OutDataTypeStr=single  RndMeth=Nearest
  Terminator : Terminator
  Trigonometric Function : Trigonometry
  Trigonometric Function1 : Trigonometry  Operator=cos
  Voltage Bias : Bias  Bias=1.5  SaturateOnIntegerOverflow=off
  abc to dq0 : spsabctodq0Lib/abc to dq0  Alignment=Aligned with phase A axis
  dq0 to abc : spsdq0toabcLib/dq0 to abc  Alignment=Aligned with phase A axis
  abc1 : Outport
  Out3 : Outport  Port=2
  T_e : Outport  Port=3
  w_m : Outport  Port=4
  wires:
  Demux1/2 -> Machine Model in DQ/2(v_q)
  Machine Model in DQ/3(th_e) -> abc to dq0/2, dq0 to abc/2, Gain6/1
  Demux1/1 -> Machine Model in DQ/1(v_d)
  Mux1/1 -> dq0 to abc/1
  Mechanical Model/1(w_m) -> w_m/1, Machine Model in DQ/3(w_m)
  Machine Model in DQ/4(T_e) -> T_e/1, Mechanical Model/1(T_e)  "Tourqe"
  Constant3/1 -> Mux1/3
  Demux1/3 -> Terminator/1
  Machine Model in DQ/1(i_d) -> Mux1/1  "i_d"
  Machine Model in DQ/2(i_q) -> Mux1/2  "i_q"
  abc to dq0/1 -> Demux1/1
  dq0 to abc/1 -> abc1/1
  abc/1 -> abc to dq0/1
  Gain6/1 -> Sum/1  "Rotor Angle"
  Constant/1 -> Sum/2
  Sum/1 -> Trigonometric Function1/1, Trigonometric Function/1  "Rotor Angle"
  Trigonometric Function/1 -> Mux/1  "Sine"
  Mux/1 -> Voltage Bias/1
  Trigonometric Function1/1 -> Mux/2  "Cos"
  Voltage Bias/1 -> Out3/1  "Sine_Cos_Voltage"

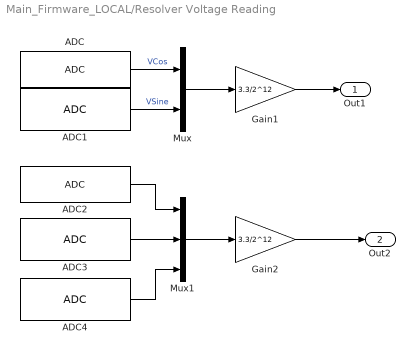
== system Main_Firmware_LOCAL/Resolver Voltage Reading ==
  ADC : c2802xlib/ADC  blkParamProc=C2000_Type5  ADCModule=B  samplingMode=Single sample mode  ADCResolution=12-bit (Single-ended input)  useSOC1=SOC0  useSOC2=SOC0_SOC1  SOCAcquisitionWindow=8  SOCTriggerSource=Software  SOCInterruptTrigger=No ADCINT  Ts=sample_time  dType=single  postInterrupt=off  interruptSel=ADCINT1  ADCINTContinuous=on  endma=off  chdma=1  conv1=ADCINA0  conv2=ADCINA0 and ADCINB0  conv1_Type4=ADCIN6  conv2_Type4=ADCIN0 and ADCIN1
      settings: LibrarySourceBlock=c28004xlib/ADC
  ADC1 : c2802xlib/ADC  blkParamProc=C2000_Type5  ADCModule=A  samplingMode=Single sample mode  ADCResolution=12-bit (Single-ended input)  useSOC1=SOC8  useSOC2=SOC0_SOC1  SOCAcquisitionWindow=8  SOCTriggerSource=Software  SOCInterruptTrigger=No ADCINT  Ts=sample_time  dType=single  postInterrupt=off  interruptSel=ADCINT1  ADCINTContinuous=on  endma=off  chdma=1  conv1=ADCINA0  conv2=ADCINA0 and ADCINB0  conv1_Type4=ADCIN6  conv2_Type4=ADCIN0 and ADCIN1
      settings: LibrarySourceBlock=c28004xlib/ADC
  ADC2 : c2802xlib/ADC  blkParamProc=C2000_Type5  ADCModule=C  samplingMode=Single sample mode  ADCResolution=12-bit (Single-ended input)  useSOC1=SOC1  useSOC2=SOC0_SOC1  SOCAcquisitionWindow=8  SOCTriggerSource=Software  SOCInterruptTrigger=No ADCINT  Ts=sample_time  dType=single  postInterrupt=off  interruptSel=ADCINT1  ADCINTContinuous=on  endma=off  chdma=1  conv1=ADCINA0  conv2=ADCINA0 and ADCINB0  conv1_Type4=ADCIN3  conv2_Type4=ADCIN0 and ADCIN1
      settings: LibrarySourceBlock=c28004xlib/ADC
  ADC3 : c2802xlib/ADC  blkParamProc=C2000_Type5  ADCModule=C  samplingMode=Single sample mode  ADCResolution=12-bit (Single-ended input)  useSOC1=SOC2  useSOC2=SOC0_SOC1  SOCAcquisitionWindow=8  SOCTriggerSource=Software  SOCInterruptTrigger=No ADCINT  Ts=sample_time  dType=single  postInterrupt=off  interruptSel=ADCINT1  ADCINTContinuous=on  endma=off  chdma=1  conv1=ADCINA0  conv2=ADCINA0 and ADCINB0  conv1_Type4=ADCIN5  conv2_Type4=ADCIN0 and ADCIN1
      settings: LibrarySourceBlock=c28004xlib/ADC
  ADC4 : c2802xlib/ADC  blkParamProc=C2000_Type5  ADCModule=A  samplingMode=Single sample mode  ADCResolution=12-bit (Single-ended input)  useSOC1=SOC3  useSOC2=SOC0_SOC1  SOCAcquisitionWindow=8  SOCTriggerSource=Software  SOCInterruptTrigger=No ADCINT  Ts=sample_time  dType=single  postInterrupt=off  interruptSel=ADCINT1  ADCINTContinuous=on  endma=off  chdma=1  conv1=ADCINA0  conv2=ADCINA0 and ADCINB0  conv1_Type4=ADCIN3  conv2_Type4=ADCIN0 and ADCIN1
      settings: LibrarySourceBlock=c28004xlib/ADC
  Gain1 : Gain  Gain=3.3/2^12  ParamDataTypeStr=single  OutDataTypeStr=single  RndMeth=Nearest
  Gain2 : Gain  Gain=3.3/2^12  ParamDataTypeStr=single  OutDataTypeStr=single  RndMeth=Nearest
  Mux : Mux  Inputs=2
  Mux1 : Mux  Inputs=3
  Out1 : Outport
  Out2 : Outport  Port=2
  wires:
  Mux/1 -> Gain1/1
  ADC/1 -> Mux/1  "VCos"
  Gain1/1 -> Out1/1
  ADC1/1 -> Mux/2  "VSine"
  Mux1/1 -> Gain2/1
  ADC2/1 -> Mux1/1
  ADC3/1 -> Mux1/2
  Gain2/1 -> Out2/1
  ADC4/1 -> Mux1/3

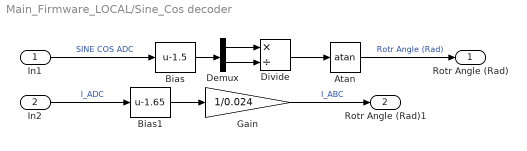
== system Main_Firmware_LOCAL/Sine_Cos decoder ==
  In1 : Inport
  In2 : Inport  Port=2
  Atan : Trigonometry  Operator=atan  OutputSignalType=real
  Bias : Bias  Bias=-1.5  SaturateOnIntegerOverflow=off
  Bias1 : Bias  Bias=-1.65  SaturateOnIntegerOverflow=off
  Demux : Demux  Outputs=2
  Divide : Product  Inputs=*/  OutMin=-3.4e38  OutMax=3.4e38  OutDataTypeStr=single  RndMeth=Nearest
  Gain : Gain  Gain=1/0.024
  Rotr Angle (Rad) : Outport
  Rotr Angle (Rad)1 : Outport  Port=2
  wires:
  Divide/1 -> Atan/1
  Demux/2 -> Divide/2
  Demux/1 -> Divide/1
  In1/1 -> Bias/1  "SINE COS ADC"
  Atan/1 -> Rotr Angle (Rad)/1  "Rotr Angle (Rad)"
  Bias/1 -> Demux/1
  In2/1 -> Bias1/1  "I_ADC"
  Bias1/1 -> Gain/1
  Gain/1 -> Rotr Angle (Rad)1/1  "I_ABC"

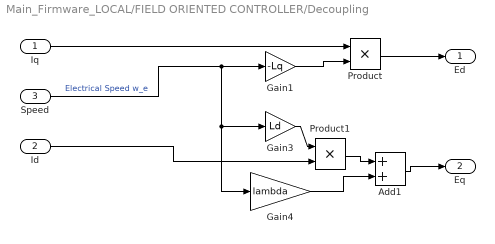
== system Main_Firmware_LOCAL/FIELD ORIENTED CONTROLLER/Decoupling ==
  Iq : Inport
  Id : Inport  Port=2
  Speed : Inport  Port=3
  Add1 : Sum  OutDataTypeStr=single  RndMeth=Nearest
  Gain1 : Gain  Gain=-Lq  ParamDataTypeStr=single  OutDataTypeStr=single  RndMeth=Nearest
  Gain3 : Gain  Gain=Ld  OutDataTypeStr=single  RndMeth=Nearest
  Gain4 : Gain  Gain=lambda  OutDataTypeStr=single  RndMeth=Nearest
  Product : Product  OutDataTypeStr=single  RndMeth=Nearest
  Product1 : Product  OutDataTypeStr=single  RndMeth=Nearest
  Ed : Outport
  Eq : Outport  Port=2
  wires:
  Product/1 -> Ed/1
  Gain3/1 -> Product1/1
  Product1/1 -> Add1/1
  Gain4/1 -> Add1/2
  Add1/1 -> Eq/1
  Speed/1 -> Gain4/1, Gain3/1, Gain1/1  "Electrical Speed w_e"
  Iq/1 -> Product/1
  Gain1/1 -> Product/2
  Id/1 -> Product1/2

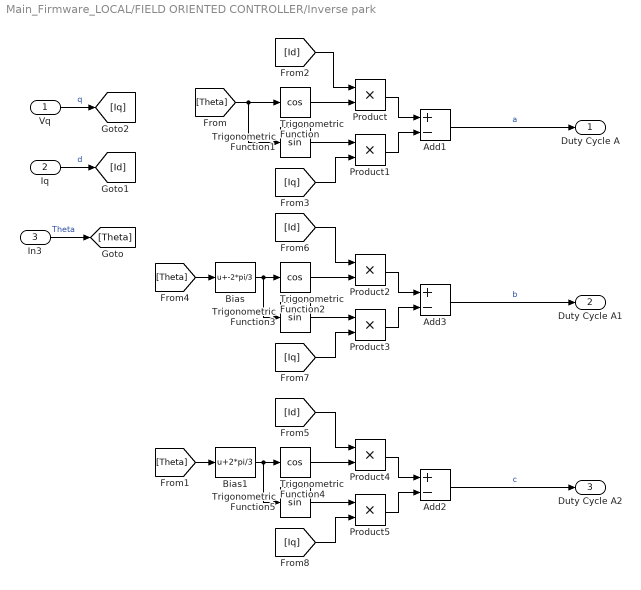
== system Main_Firmware_LOCAL/FIELD ORIENTED CONTROLLER/Inverse park ==
  Vq : Inport
  Iq : Inport  Port=2
  In3 : Inport  Port=3
  Add1 : Sum  Inputs=+-  OutDataTypeStr=single  RndMeth=Nearest
  Add2 : Sum  Inputs=+-  OutDataTypeStr=single  RndMeth=Nearest
  Add3 : Sum  Inputs=+-  OutDataTypeStr=single  RndMeth=Nearest
  Bias : Bias  Bias=-2*pi/3  SaturateOnIntegerOverflow=off
  Bias1 : Bias  Bias=2*pi/3  SaturateOnIntegerOverflow=off
  Product{,1..5} (6 alike) : Product  OutDataTypeStr=single  RndMeth=Nearest
  Trigonometric Function : Trigonometry  Operator=cos
  Trigonometric Function1 : Trigonometry
  Trigonometric Function2 : Trigonometry  Operator=cos
  Trigonometric Function3 : Trigonometry
  Trigonometric Function4 : Trigonometry  Operator=cos
  Trigonometric Function5 : Trigonometry
  Duty Cycle A : Outport
  Duty Cycle A1 : Outport  Port=2
  Duty Cycle A2 : Outport  Port=3
  wires:
  Iq/1 -> [Id]  "d"
  Vq/1 -> [Iq]  "q"
  Add1/1 -> Duty Cycle A/1  "a"
  Add3/1 -> Duty Cycle A1/1  "b"
  In3/1 -> [Theta]  "Theta"
  [Theta] -> Trigonometric Function1/1, Trigonometric Function/1
  [Iq] -> Product1/2
  Trigonometric Function/1 -> Product/2
  [Id] -> Product/1
  Trigonometric Function1/1 -> Product1/1
  Product/1 -> Add1/1
  Product1/1 -> Add1/2
  Product3/1 -> Add3/2
  [Theta] -> Bias/1
  [Id] -> Product2/1
  Product2/1 -> Add3/1
  Trigonometric Function3/1 -> Product3/1
  [Iq] -> Product3/2
  Trigonometric Function2/1 -> Product2/2
  Bias/1 -> Trigonometric Function3/1, Trigonometric Function2/1
  Trigonometric Function4/1 -> Product4/2
  [Id] -> Product4/1
  [Theta] -> Bias1/1
  [Iq] -> Product5/2
  Add2/1 -> Duty Cycle A2/1  "c"
  Product5/1 -> Add2/2
  Trigonometric Function5/1 -> Product5/1
  Product4/1 -> Add2/1
  Bias1/1 -> Trigonometric Function5/1, Trigonometric Function4/1

== system Main_Firmware_LOCAL/FIELD ORIENTED CONTROLLER/Speed Calc ==
  U : Inport
  Discrete Derivative calc2 : simulink/Discrete/Discrete Derivative  gainval=1.0  ICPrevScaledInput=0.0  OutMin=[]  OutMax=[]  OutDataTypeStr=single  OutputDataTypeScalingMode=single  OutDataType=fixdt(1, 16)  OutScaling=2^-10  RndMeth=Nearest  DoSatur=off
  Ignore Overflow : Subsystem
  Out1 : Outport
  wires:
  Discrete Derivative calc2/1 -> Ignore Overflow/1(In2)  "Electrical speed (Rad/s)"
  U/1 -> Discrete Derivative calc2/1
  Ignore Overflow/1(Out1) -> Out1/1  "W_e"

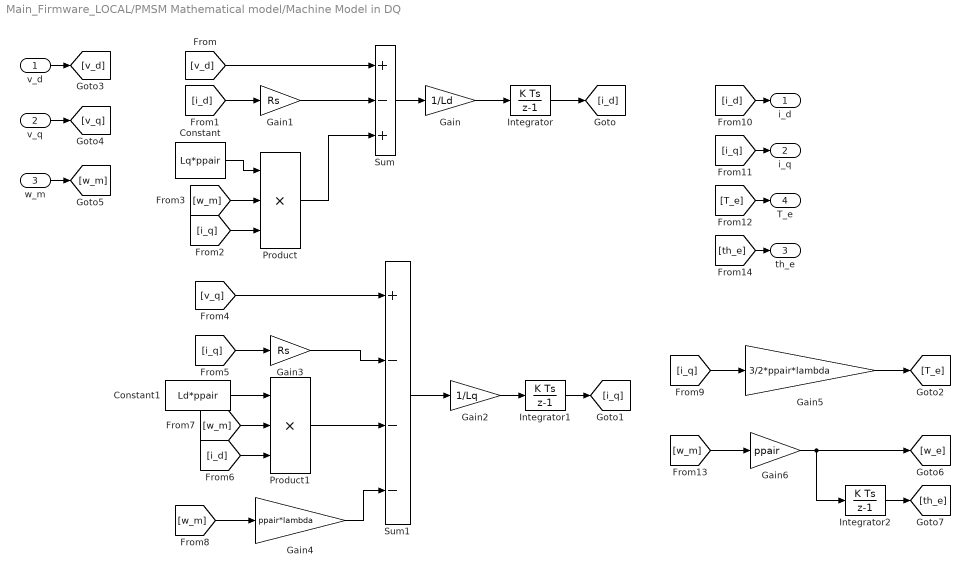
== system Main_Firmware_LOCAL/PMSM Mathematical model/Machine Model in DQ ==
  v_d : Inport
  v_q : Inport  Port=2
  w_m : Inport  Port=3
  Constant : Constant  Value=Lq*ppair  OutDataTypeStr=single
  Constant1 : Constant  Value=Ld*ppair  OutDataTypeStr=single
  Gain : Gain  Gain=1/Ld
  Gain1 : Gain  Gain=Rs  OutDataTypeStr=single  RndMeth=Nearest
  Gain2 : Gain  Gain=1/Lq
  Gain3 : Gain  Gain=Rs  OutDataTypeStr=single  RndMeth=Nearest
  Gain4 : Gain  Gain=ppair*lambda  ParamDataTypeStr=single
  Gain5 : Gain  Gain=3/2*ppair*lambda  OutDataTypeStr=single  RndMeth=Nearest
  Gain6 : Gain  Gain=ppair  OutDataTypeStr=single  RndMeth=Nearest
  Integrator : DiscreteIntegrator  SampleTime=0.000100000000000000005  LimitOutput=on  UpperSaturationLimit=3.40282347E+38  LowerSaturationLimit=-3.40282347E+38  ICPrevOutput=DiscIntNeverNeededParam  ICPrevScaledInput=DiscIntNeverNeededParam  mask(DiscretizedDiscreteIntegrator){}
      mask init:
      | %zoh
  Integrator1 : DiscreteIntegrator  SampleTime=-1  LimitOutput=on  UpperSaturationLimit=3.40282347E+38  LowerSaturationLimit=-3.40282347E+38  ICPrevOutput=DiscIntNeverNeededParam  ICPrevScaledInput=DiscIntNeverNeededParam  mask(DiscretizedDiscreteIntegrator){}
      mask init:
      | %zoh
  Integrator2 : DiscreteIntegrator  SampleTime=-1  LimitOutput=on  UpperSaturationLimit=3.40282347E+38  LowerSaturationLimit=-3.40282347E+38  ICPrevOutput=DiscIntNeverNeededParam  ICPrevScaledInput=DiscIntNeverNeededParam  mask(DiscretizedDiscreteIntegrator){}
      mask init:
      | %zoh
  Product : Product  Inputs=3  OutDataTypeStr=single  RndMeth=Nearest
  Product1 : Product  Inputs=3  OutDataTypeStr=single  RndMeth=Nearest
  Sum : Sum  Inputs=+-+  OutDataTypeStr=single  RndMeth=Nearest
  Sum1 : Sum  Inputs=+---  OutDataTypeStr=single  RndMeth=Nearest
  i_d : Outport
  i_q : Outport  Port=2
  th_e : Outport  Port=3
  T_e : Outport  Port=4
  wires:
  Constant/1 -> Product/1
  Product/1 -> Sum/3
  Integrator/1 -> [i_d]
  [v_d] -> Sum/1
  [w_m] -> Product1/2
  Gain4/1 -> Sum1/4
  [i_q] -> Product/3
  Sum/1 -> Gain/1
  [w_m] -> Gain4/1
  [i_d] -> Gain1/1
  Sum1/1 -> Gain2/1
  Gain/1 -> Integrator/1
  Gain5/1 -> [T_e]
  [i_q] -> Gain5/1
  Gain1/1 -> Sum/2
  Integrator1/1 -> [i_q]
  [i_q] -> Gain3/1
  Product1/1 -> Sum1/3
  Constant1/1 -> Product1/1
  Gain2/1 -> Integrator1/1
  [v_q] -> Sum1/1
  Gain3/1 -> Sum1/2
  [i_d] -> Product1/3
  [w_m] -> Product/2
  v_d/1 -> [v_d]
  v_q/1 -> [v_q]
  [i_d] -> i_d/1
  [i_q] -> i_q/1
  [T_e] -> T_e/1
  w_m/1 -> [w_m]
  [w_m] -> Gain6/1
  Gain6/1 -> Integrator2/1, [w_e]
  Integrator2/1 -> [th_e]
  [th_e] -> th_e/1
